simulink model ""  (R2025b)
settings: Solver=VariableStepAuto  StartTime=0.0  StopTime=inf  RelTol=1e-3
libraries: instrumentseriallib x3, etargetslib x1, svdutilitieslib x1
settings Model: Creator=erik  LastModifiedBy=erik

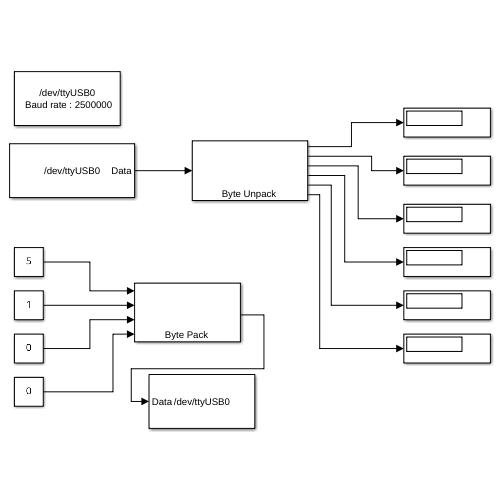
[thumbnail: Simulink's stored preview of the top-level diagram]
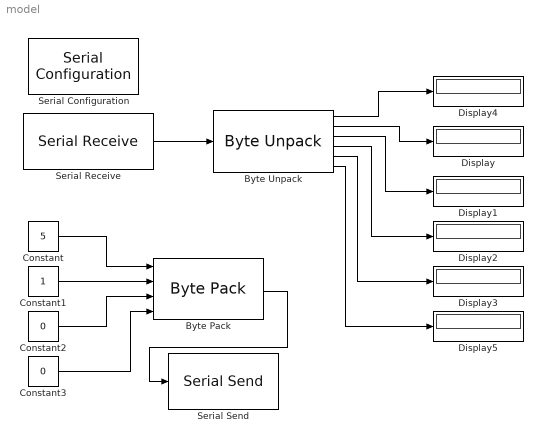
== system model ==
  Byte Pack : etargetslib/Byte Pack  datatypes={'single','boolean','boolean','single'}  byteAlign=1
  Byte Unpack : svdutilitieslib/Byte Unpack  dimensions={[1],[1],[1],[1],[1],[1]}  datatypes={'uint8', 'uint8','uint8','uint8','uint8','uint8'}  byteAlign=1  blockPlatform=tic2000
      settings: LibrarySourceBlock=c2000lib/Target Communication/Byte Unpack
  Constant : Constant  Value=5  OutDataTypeStr=single
  Constant1 : Constant  OutDataTypeStr=boolean
  Constant2 : Constant  Value=0  OutDataTypeStr=boolean
  Constant3 : Constant  Value=0  OutDataTypeStr=single
  Display{,1..5} (6 alike) : Display
  Serial Configuration : instrumentseriallib/Serial Configuration  Priority=-200000  PortSel=/dev/ttyUSB0  Port=/dev/ttyUSB0  ComPort=/dev/ttyUSB0  BaudRate=2500000  DataBits=8  Parity=none  StopBits=1  ByteOrder=little-endian  FlowControl=none  Timeout=10  SimulateUsing=Interpreted execution  BlockInModel=on  aMode=1
      settings: LibrarySourceBlock=embeddedtargetslib/Host Communication/Serial Configuration
  Serial Receive : instrumentseriallib/Serial Receive  Priority=1  PortSel=/dev/ttyUSB0  Port=/dev/ttyUSB0  ComPort=/dev/ttyUSB0  DataType=uint8  SaveDataType=uint8  ToggleHeader=off  Header=[]  ToggleDataSize=on  DataSize=[6 1]  ToggleTerminator=off  Terminator=<none>  CustomTerminator=[]  InputFormat=Column major  EnableBlockingMode=on  ActionDataUnavailable=Output last received value  ActionWhenDataUnavailable=Output last received value  CustomValue=0  SampleTime=0.01  SimulateUsing=Interpreted execution  BlockInModel=on  aMode=1  LibraryInUse=c2000lib
      settings: LibrarySourceBlock=c2000lib/Host Communication/Serial Receive
  Serial Send : instrumentseriallib/Serial Send  Priority=1  PortSel=/dev/ttyUSB0  Port=/dev/ttyUSB0  ComPort=/dev/ttyUSB0  Header=[]  Terminator=<none>  CustomTerminator=[]  EnableBlockingMode=on  SimulateUsing=Interpreted execution  BlockInModel=on  aMode=1
      settings: LibrarySourceBlock=embeddedtargetslib/Host Communication/Serial Send
  wires:
  Serial Receive/1 -> Byte Unpack/1
  Byte Unpack/1 -> Display4/1
  Byte Unpack/2 -> Display/1
  Byte Pack/1 -> Serial Send/1
  Constant/1 -> Byte Pack/1
  Constant1/1 -> Byte Pack/2
  Constant2/1 -> Byte Pack/3
  Constant3/1 -> Byte Pack/4
  Byte Unpack/3 -> Display1/1
  Byte Unpack/4 -> Display2/1
  Byte Unpack/5 -> Display3/1
  Byte Unpack/6 -> Display5/1
